simulink model "mpc_pendcartPlant"  (R2019a)
settings: Solver=ode45  StartTime=0.0  StopTime=10.0  RelTol=1e-3  EnableMultiTasking=on
values from neighbouring files (symbols this model uses):
  f = 1    [ControlOfAnInvertedPendulumOnACartExample.m]
  J = 1    [ControlOfAnInvertedPendulumOnACartExample.m]
  l = 0.45    [ControlOfAnInvertedPendulumOnACartExample.m]
  m_p = 0.853    [ControlOfAnInvertedPendulumOnACartExample.m]
settings Model: Creator=The MathWorks, Inc.  LastModifiedBy=Lucifer
settings SolverCC: MinimalZcImpactIntegration=on
settings DataIOCC: LimitDataPoints=on  ReturnWorkspaceOutputs=off
settings OptimizationCC: LifeSpan=inf
settings DebuggingCC: AllowSymbolicDim=off  PregeneratedLibrarySubsystemCodeDiagnostic=none  SFUnexpectedBacktrackingDiag=warning  SFNoUnconditionalDefaultTransitionDiag=warning  SFExecutionAtInitializationDiag=none  ArithmeticOperatorsInVariantConditions=warning
settings ModelReferenceCC: PropagateSignalLabelsOutOfModel=off
settings SFSimCC: SimUseLocalCustomCode=off
settings RTWCC: RTWUseLocalCustomCode=off
settings CodeAppCC: StateflowObjectComments=on
settings GRTTargetCC: TargetLangStandard=C89/C90 (ANSI)
settings ConfigComp: CovScope=ReferencedModels  CovMetricSettings=dw  CovHtmlReporting=on  CovSaveCumulativeToWorkspaceVar=on  CovSaveSingleToWorkspaceVar=on  CovExternalEMLEnable=off
settings SimscapeCC: SimscapeNormalizeSystem=off

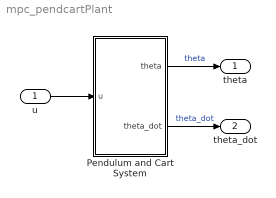
== system mpc_pendcartPlant ==
  u : Inport
  Pendulum and Cart System : Subsystem  mask{mCartPara=1, mPendPara=1, gPara=9.81, LPara=0.5, KdPara=10}
      mask prompts: mCartPara "Mass of Cart"; mPendPara "Mass of Pendulum"; gPara "Gravity"; LPara "Length of Pendulum"; KdPara "Friction coefficient of Cart"
      mask help: Pendulum and Cart System
      mask init:
      | mCart = str2double(get_param(gcb,'mCartPara'));
      | mPend = str2double(get_param(gcb,'mPendPara'));
      | g = str2double(get_param(gcb,'gPara'));
      | L = str2double(get_param(gcb,'LPara'));
      | Kd = str2double(get_param(gcb,'KdPara'));
  theta : Outport
  theta_dot : Outport  Port=2
  wires:
  Pendulum and Cart System/1(theta) -> theta/1  "theta"
  Pendulum and Cart System/2(theta_dot) -> theta_dot/1  "theta_dot"
  u/1 -> Pendulum and Cart System/1(u)

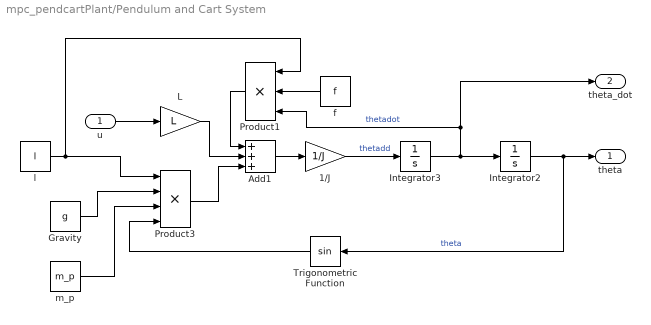
== system mpc_pendcartPlant/Pendulum and Cart System ==
  u : Inport
  1/J : Gain  Gain=1/J
  Add1 : Sum  Inputs=+++
  Gravity : Constant  Value=g
  Integrator2 : Integrator  ContinuousStateAttributes='theta'
  Integrator3 : Integrator  ContinuousStateAttributes='thetadot'
  L : Gain  Gain=L
  Product1 : Product  Inputs=3
  Product3 : Product  Inputs=4
  Trigonometric Function : Trigonometry
  f : Constant  Value=f
  l : Constant  Value=l
  m_p : Constant  Value=m_p
  theta : Outport
  theta_dot : Outport  Port=2
  wires:
  1/J/1 -> Integrator3/1  "thetadd"
  Product3/1 -> Add1/3
  Integrator3/1 -> Integrator2/1, Product1/3, theta_dot/1  "thetadot"
  Integrator2/1 -> Trigonometric Function/1, theta/1  "theta"
  Add1/1 -> 1/J/1
  L/1 -> Add1/2
  u/1 -> L/1
  l/1 -> Product1/1, Product3/1
  Gravity/1 -> Product3/2
  m_p/1 -> Product3/3
  Trigonometric Function/1 -> Product3/4
  f/1 -> Product1/2
  Product1/1 -> Add1/1
